simulink model "suspension"  (R2024a)
settings: Solver=VariableStepAuto  StartTime=0.0  StopTime=10.0  MaxStep=0.01  RelTol=1e-3
PreLoadFcn:
  | m = 2;
  | k = 5;
  | c = 3;
settings Model: Creator=The MathWorks, Inc.  LastModifiedBy=grouleau
settings SolverCC: AlgebraicLoopSolver=TrustRegion
settings DataIOCC: ExternalInput=[0 1]  LoadExternalInput=on
settings OptimizationCC: ReuseModelBlockBuffer=off
settings DebuggingCC: UnconnectedInputMsg=warning  UnconnectedOutputMsg=warning  UnconnectedLineMsg=warning  PregeneratedLibrarySubsystemCodeDiagnostic=none  ArithmeticOperatorsInVariantConditions=warning
settings ModelReferenceCC: EnableRefExpFcnMdlSchedulingChecks=on
settings SFSimCC: SimUseLocalCustomCode=off  CustomCodeUndefinedFunction=UseInterfaceOnly
settings RTWCC: RTWUseLocalCustomCode=off  GPUComputeCapability=3.5

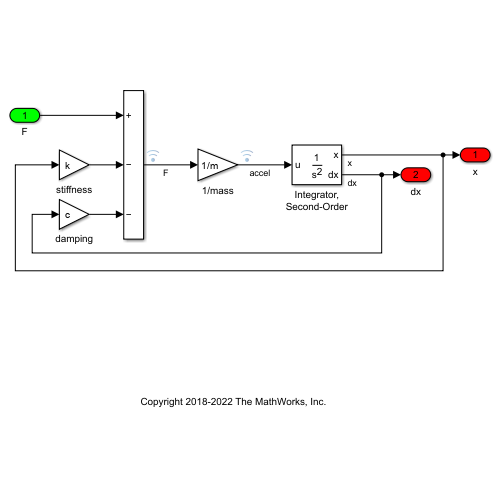
[thumbnail: Simulink's stored preview of the top-level diagram]
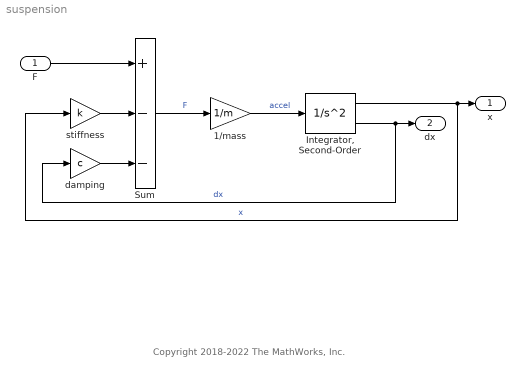
== system suspension ==
  note: Copyright 2018-2022 The MathWorks, Inc.
  F : Inport
  1/mass : Gain  Gain=1/m
  "Integrator, Second-Order" : SecondOrderIntegrator
  Sum : Sum  Inputs=+--
  damping : Gain  Gain=c
  stiffness : Gain  Gain=k
  x : Outport
  dx : Outport  Port=2
  wires:
  F/1 -> Sum/1
  damping/1 -> Sum/3
  stiffness/1 -> Sum/2
  Sum/1 -> 1/mass/1  "F"
  "Integrator, Second-Order"/2 -> dx/1, damping/1  "dx"
  "Integrator, Second-Order"/1 -> x/1, stiffness/1  "x"
  1/mass/1 -> "Integrator, Second-Order"/1  "accel"
